simulink model "ADCPlayground"  (R2024b)
settings: Solver=FixedStepAuto  StartTime=0.0  StopTime=inf  RelTol=1e-3  EnableMultiTasking=on
libraries: bbblueBasicLib x1
settings Model: ExtModeTrigDuration=100  Creator=Henrik  LastModifiedBy=Henrik
settings SolverCC: PositivePriorityOrder=on
settings OptimizationCC: DefaultParameterBehavior=Inlined  EnhancedBackFolding=on  PassReuseOutputArgsAs=Individual arguments  ZeroExternalMemoryAtStartup=off  ZeroInternalMemoryAtStartup=off  MaxStackSize=64  OptimizeBlockOrder=speed  DifferentSizesBufferReuse=on  OptimizationCustomize=off  EfficientTunableParamExpr=on
settings DebuggingCC: ParameterTunabilityLossMsg=error
settings HardwareCC: ProdBitPerPointer=32  ProdBitPerSizeT=32  ProdBitPerPtrDiffT=32  ProdLargestAtomicInteger=Long  ProdLargestAtomicFloat=Double  ProdWordSize=32  ProdHWDeviceType=ARM Compatible->ARM Cortex-A (32-bit)  UseEmbeddedCoderFeatures=off
settings SFSimCC: MATLABDynamicMemAlloc=off
settings RTWCC: Description=Embedded Coder  SystemTargetFile=ert.tlc  HardwareBoard=BeagleBone Blue  TLCOptions="-aInlineSetEventsForThisBaseRateFcn=TLC_FALSE -aSuppressMultiTaskScheduler=TLC_FALSE  -aRateBasedStepFcn=0"  TemplateMakefile=ert_default_tmf  Toolchain=GNU GCC BeagleBone Blue
settings CodeAppCC: ForceParamTrailComments=on  IgnoreCustomStorageClasses=off  OperatorAnnotations=on  SimulinkDataObjDesc=on  SFDataObjDesc=on  InsertBlockDesc=on
settings ERTTargetCC: SupportNonInlinedSFcns=on  SupportVariableSizeSignals=on

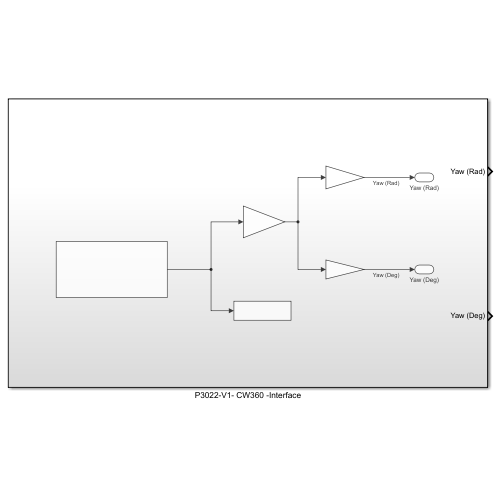
[thumbnail: Simulink's stored preview of the top-level diagram]
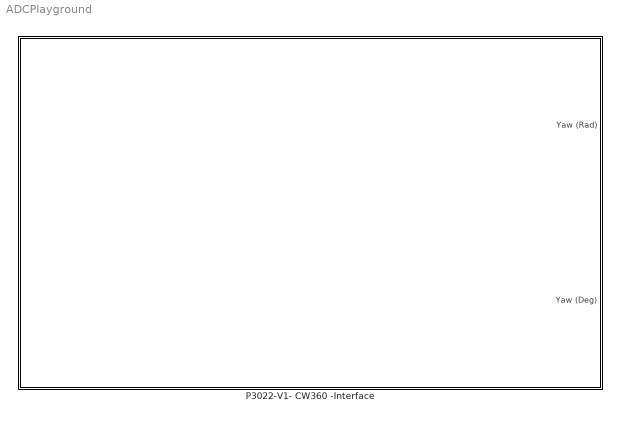
== system ADCPlayground ==
  P3022-V1- CW360 -Interface : Subsystem

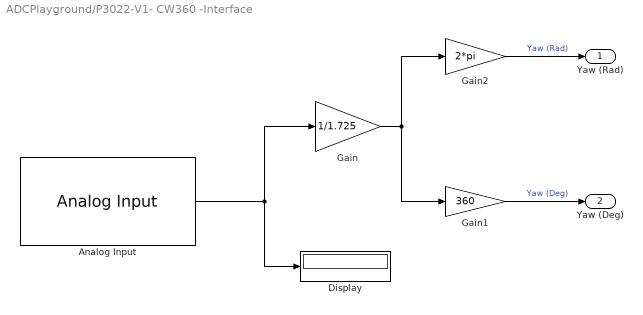
== system ADCPlayground/P3022-V1- CW360 -Interface ==
  Analog Input : bbblueBasicLib/Analog Input  Pin=AIN0  Mode=Volt  SampleTime=0.1  SimulateUsing=Code generation
  Display : Display
  Gain : Gain  Gain=1/1.725
  Gain1 : Gain  Gain=360
  Gain2 : Gain  Gain=2*pi
  Yaw (Rad) : Outport
  Yaw (Deg) : Outport  Port=2
  wires:
  Gain/1 -> Gain2/1, Gain1/1
  Analog Input/1 -> Gain/1, Display/1
  Gain2/1 -> Yaw (Rad)/1  "Yaw (Rad)"
  Gain1/1 -> Yaw (Deg)/1  "Yaw (Deg)"
